simulink model "trapecio_simulink"  (R2025a)
settings: Solver=VariableStepAuto  StartTime=0.0  StopTime=10.0  RelTol=1e-3
settings Model: Creator=nicoditeodoro  LastModifiedBy=nicoditeodoro

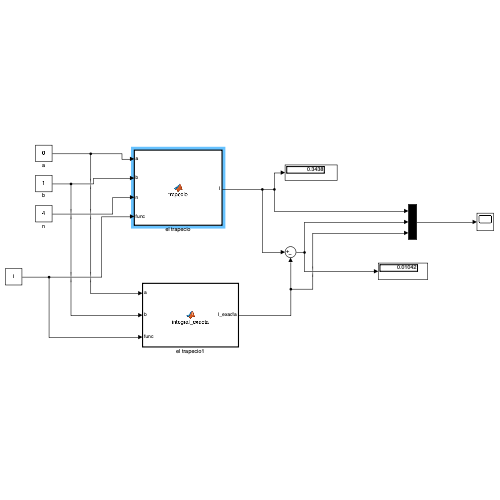
[thumbnail: Simulink's stored preview of the top-level diagram]
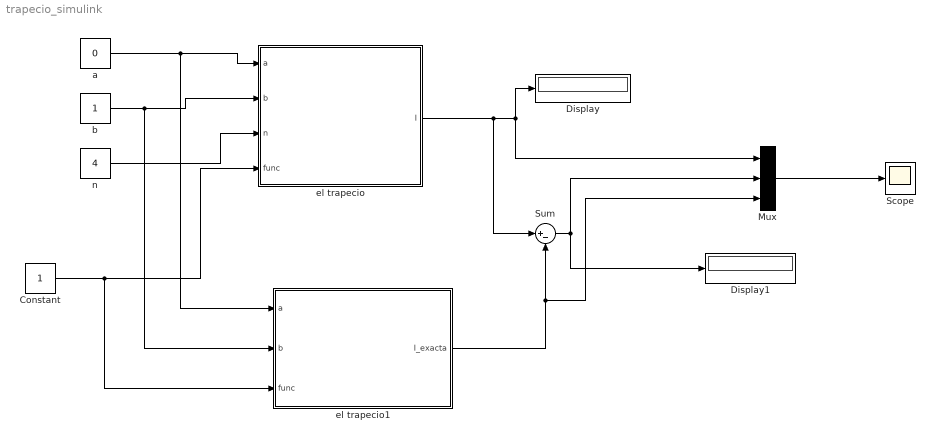
== system trapecio_simulink ==
  Constant : Constant
  Display : Display
  Display1 : Display
  Mux : Mux  Inputs=3
  Scope : Scope
      settings: TimeSpan=10  ActiveDisplayYMinimum=-0.031249999999999972  ActiveDisplayYMaximum=0.38541666666666669
  Sum : Sum  Inputs=|+-
  a : Constant  Value=0
  b : Constant
  el trapecio : MATLAB Function  TreatAsAtomicUnit=on
  el trapecio1 : MATLAB Function  TreatAsAtomicUnit=on
  n : Constant  Value=4
  wires:
  Constant/1 -> el trapecio1/3(func), el trapecio/4(func)
  a/1 -> el trapecio1/1(a), el trapecio/1(a)
  b/1 -> el trapecio1/2(b), el trapecio/2(b)
  n/1 -> el trapecio/3(n)
  el trapecio/1(I) -> Sum/1, Mux/1, Display/1
  el trapecio1/1(I_exacta) -> Mux/3, Sum/2
  Sum/1 -> Mux/2, Display1/1
  Mux/1 -> Scope/1

== matlab function trapecio_simulink/el trapecio ==
  data: a input; b input; n input; func input; I output
function I = trapecio(a,b,n,func)

I = 0;         
n = round(n);   

h = (b-a)/n;
x = linspace(a,b,n+1);

y = zeros(size(x));

for i = 1:length(x)
    if func == 1
        y(i) = x(i)^2;
    elseif func == 2
        y(i) = sin(x(i));
    elseif func == 3
        y(i) = exp(x(i));
    else
        y(i) = 0;
    end
end

I = h*( sum(y) - 0.5*(y(1)+y(end)) );

== matlab function trapecio_simulink/el trapecio1 ==
  data: a input; b input; func input; I_exacta output
function I_exacta = integral_exacta(a,b,func)

I_exacta = 0;   

if func == 1
    % Integral de x^2
    I_exacta = (b^3 - a^3)/3;

elseif func == 2
    % Integral de sin(x)
    I_exacta = -cos(b) + cos(a);

elseif func == 3
    % Integral de e^x
    I_exacta = exp(b) - exp(a);

else
    I_exacta = 0;  
end
